simulink model "FM_ModulatorandDemodulator"  (R2021a)
settings: Solver=VariableStepAuto  StartTime=0.0  StopTime=10.0  RelTol=1e-3
libraries: commsynccomp2 x2, dspfdesign x1
settings Model: Creator=ZephyrY  LastModifiedBy=ZephyrY

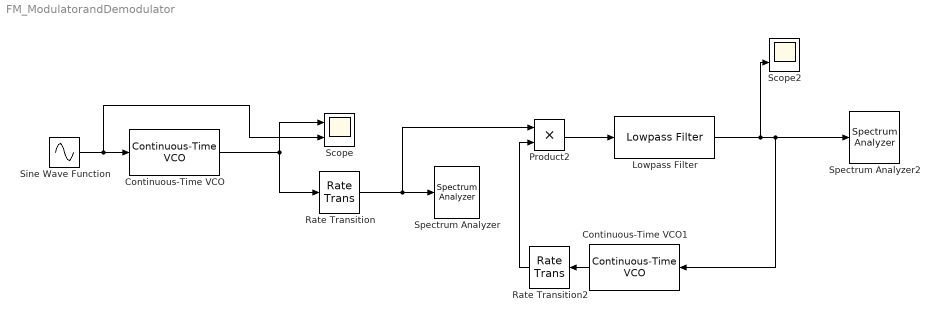
== system FM_ModulatorandDemodulator ==
  Continuous-Time VCO : commsynccomp2/Continuous-Time VCO  Ac=4  Fc=100  Kc=2  Ph=0
      settings: SourceProductBaseCode=CM
  Continuous-Time VCO1 : commsynccomp2/Continuous-Time VCO  Ac=4  Fc=100  Kc=2  Ph=0
      settings: SourceProductBaseCode=CM
  Lowpass Filter : dspfdesign/Lowpass Filter  FilterType=FIR  DesignForMinimumOrder=off  FilterOrder=200  PassbandFrequency=28  StopbandFrequency=30  PassbandRipple=0.1  StopbandAttenuation=99  InheritSampleRate=on  SampleRate=44100  SimulateUsing=Interpreted execution  roundingMode=Floor  coeffsDataTypeStr=fixdt(1,16)
  Product2 : Product
  Rate Transition : RateTransition  OutPortSampleTime=1e-4
  Rate Transition2 : RateTransition  OutPortSampleTime=1e-4
  Scope : Scope  NumInputPorts=2
  Scope2 : Scope  NumInputPorts=2
  Sine Wave Function : Sin  Amplitude=2  Frequency=2*pi*10  Phase=pi/2  SampleTime=1e-4
  Spectrum Analyzer : SpectrumAnalyzer
  Spectrum Analyzer2 : SpectrumAnalyzer
  wires:
  Sine Wave Function/1 -> Scope/2, Continuous-Time VCO/1
  Continuous-Time VCO/1 -> Scope/1, Rate Transition/1
  Rate Transition/1 -> Product2/1, Spectrum Analyzer/1
  Rate Transition2/1 -> Product2/2
  Product2/1 -> Lowpass Filter/1
  Continuous-Time VCO1/1 -> Rate Transition2/1
  Lowpass Filter/1 -> Scope2/2, Continuous-Time VCO1/1, Spectrum Analyzer2/1
